simulink model "playground"  (R2024a)
settings: Solver=VariableStepAuto  StartTime=0.0  StopTime=10.0  RelTol=1e-3
InitFcn:
  | a = 0.672; % M + ma/2 + mb, kg
  | b = 0.0051; % (ma/2 + mb)*L, kg*m
  | % c = 0.0021; % (ma/4 + mb)*L^2 + I, kg*m^2
  | g = 9.81;
  | u = 1;
  | 
  | T1 = 0.2;
  | T2 = 0.1;
  | Tf = 0.05;
  | 
  | x1 = 0;
  | x2 = 0;
  | x3 = 0;
  | x4 = 0;
  | x1p = 0;
  | x2p = 0;
  | x3p = 0;
  | x4p = 0;
  | 
  | r = 1;
  | 
  | b0 = 1;
  | A = [0 1 0;
  |      0 0 1;
  |      0 0 0];
  | b_ = [0; b0; 0];
  | c = [1; 0; 0];
  | 
  | % A_CP = [0 1;
  | %        0 0];
  | %
  | % b_CP = [0; 1];
  | %
  | % w_CL = 70;
  | %
  | % k = place(A_CP', b_CP, -w_CL*[1 1.01])';
  | %
  | % k_ESO = 0.9;
  | %
  | % l = place(A',c,-w_CL*k_ESO*[0.99,1,1.01])';
  | 
  | % k_ESO = 10;
  | 
  | % wc_ = 70;
  | % Kx_ = place(A',b_,-wc_*[1 1])';
  | %
  | % k = [5;5];
  | %
  | % w0 = 60;
  | % l = place(A',c,-w0*[0.99,1,1.01])';
  | 
  | %% Liczenie k
  | w_CL = 5;
  | n=2;
  | k = zeros(n,1);
  | for i = 1:n
  |     k(i) = ((factorial(n))/(factorial(n-i+1)*factorial(i-1)))*w_CL^(n-i+1);
  | end
  | 
  | k_r = [k(2); 1];
  | 
  | %% Liczenie l
  | k_ESO = 50;
  | l = zeros(n+1,1);
  | 
  | for i = 1:n+1
  |     l(i) = (factorial(n+1)/(factorial(n-i+1)*factorial(i)))*(k_ESO)^(i);
  | end
  | 
  | % %% PRZYPISANIE POSZCZEGÓLNYCH L:
  | % l1 = l(1);
  | % l2 = l(2);
  | % %% OKREŚLENIE BETY:
  | % B1 = 3 * k_ESO;
  | % B2 = 3 * k_ESO^2;
  | % B3 = k_ESO^3;
  | 
  | %% W ARTYKULE MADONSKI K,L ODPOWIADA L I B W ARTYKULE JIN H.
  | l1 = k(2);
  | l2 = k(1);
  | 
  | B1 = l(1);
  | B2 = l(2);
  | B3 = l(3);
  | 
  | %% WYZNACZENIE PARAMETRÓW:
  | Kc = (B2 * l2 + B3 * l1)/(b0*(B1 * l1 + B2 + l2));
  | tau_i = (B2 * l2 + B3 * l1)/(B3 * l2);
  | tau_d = (B1 * l2 + B2 * l1 + B3)/(B2 * l2 + B3 * l1);
  | wl = sqrt(B1 * l1 + B2 + l2);
  | zeta_l = (B1 + l1)/(2*sqrt(B1 * l1 + B2 + l2));
  | %% Wzmocnienia regulatora CPID:
  | Kp = Kc;
  | Ki = Kc/tau_i;
  | Kd = Kc * tau_d;
  | 
  | %% NOWE NASTAWY PID
  | % Kp = (k(1)*l(1)+k(2)*l(3))/(b0*(k(2)*l(1)+l(2)+k(1)));
  | % Ki = (k(1)*l(3))/(b0*(k(2)*l(1)+l(2)+k(1)));
  | % Kd = (k(1)*l(1)+k(2)*l(2)+l(3))/(b0*(k(2)*l(1)+l(2)+k(1)));
settings Model: Creator=kubat  LastModifiedBy=kubat

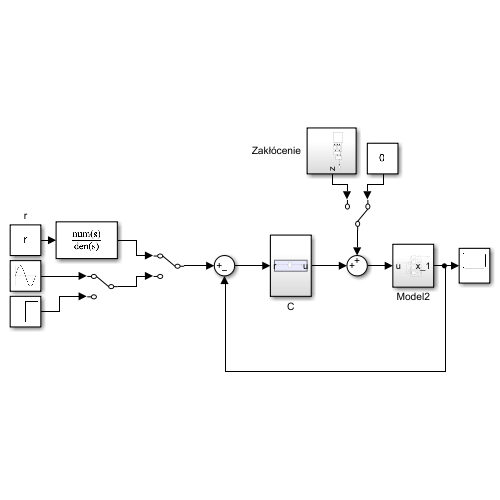
[thumbnail: Simulink's stored preview of the top-level diagram]
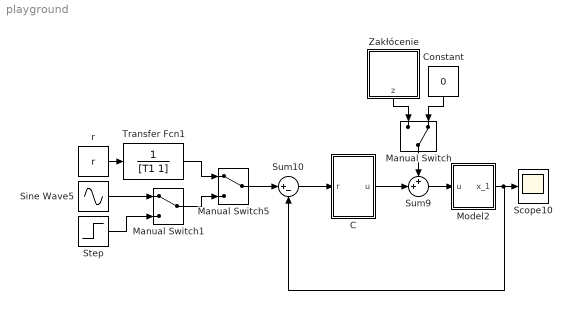
== system playground ==
  C : Subsystem
  Constant : Constant  Value=0
  Manual Switch : ManualSwitch  CurrentSetting=0
  Manual Switch1 : ManualSwitch
  Manual Switch5 : ManualSwitch
  Model2 : Subsystem
  Scope10 : Scope
  Sine Wave5 : Sin  Amplitude=u  SampleTime=0
  Step : Step  After=r  SampleTime=0
  Sum10 : Sum  Inputs=|+-
  Sum9 : Sum  Inputs=++|
  Transfer Fcn1 : TransferFcn  Denominator=[T1 1]
  Zakłócenie : Subsystem
  r : Constant  Value=r
  wires:
  Sum10/1 -> C/1(r)
  Sum9/1 -> Model2/1(u)
  Manual Switch1/1 -> Manual Switch5/2
  Sine Wave5/1 -> Manual Switch1/1
  r/1 -> Transfer Fcn1/1
  Manual Switch5/1 -> Sum10/1
  C/1(u) -> Sum9/2
  Transfer Fcn1/1 -> Manual Switch5/1
  Step/1 -> Manual Switch1/2
  Model2/1(x_1) -> Sum10/2, Scope10/1
  Constant/1 -> Manual Switch/2
  Zakłócenie/1(z) -> Manual Switch/1
  Manual Switch/1 -> Sum9/1

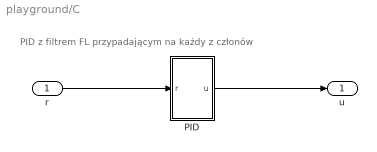
== system playground/C ==
  note: PID z filtrem FL przypadającym na każdy z członów
  r : Inport
  PID : Subsystem
  u : Outport
  wires:
  r/1 -> PID/1(r)
  PID/1(u) -> u/1

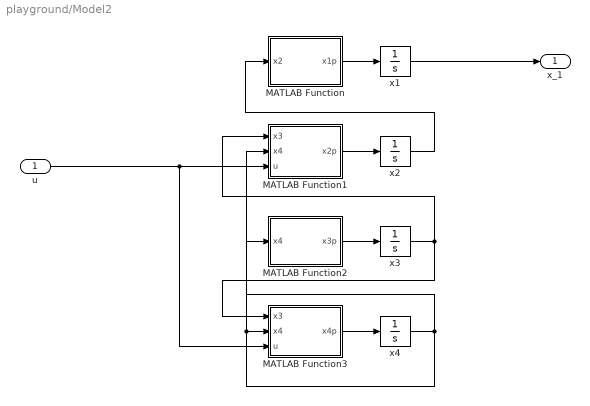
== system playground/Model2 ==
  u : Inport
  MATLAB Function : MATLAB Function  TreatAsAtomicUnit=on
  MATLAB Function1 : MATLAB Function  TreatAsAtomicUnit=on
  MATLAB Function2 : MATLAB Function  TreatAsAtomicUnit=on
  MATLAB Function3 : MATLAB Function  TreatAsAtomicUnit=on
  x{1..4} (4 alike) : Integrator
  x_1 : Outport
  wires:
  u/1 -> MATLAB Function3/3(u), MATLAB Function1/3(u)
  x4/1 -> MATLAB Function2/1(x4), MATLAB Function3/2(x4), MATLAB Function1/2(x4)
  MATLAB Function/1(x1p) -> x1/1
  x3/1 -> MATLAB Function1/1(x3), MATLAB Function3/1(x3)
  x2/1 -> MATLAB Function/1(x2)
  MATLAB Function2/1(x3p) -> x3/1
  MATLAB Function1/1(x2p) -> x2/1
  MATLAB Function3/1(x4p) -> x4/1
  x1/1 -> x_1/1

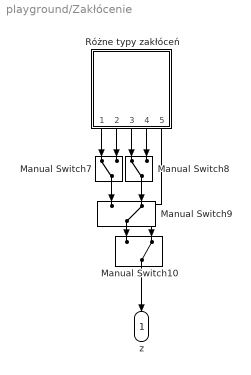
== system playground/Zakłócenie ==
  Manual Switch10 : ManualSwitch  CurrentSetting=0
  Manual Switch7 : ManualSwitch
  Manual Switch8 : ManualSwitch
  Manual Switch9 : ManualSwitch  CurrentSetting=0
  Różne typy zakłóceń : Subsystem
  z : Outport
  wires:
  Manual Switch10/1 -> z/1
  Manual Switch9/1 -> Manual Switch10/1
  Różne typy zakłóceń/2(Const.2) -> Manual Switch7/2
  Różne typy zakłóceń/5(PWM) -> Manual Switch10/2
  Różne typy zakłóceń/4(nSin.) -> Manual Switch8/2
  Różne typy zakłóceń/1(Const.1) -> Manual Switch7/1
  Manual Switch8/1 -> Manual Switch9/2
  Manual Switch7/1 -> Manual Switch9/1
  Różne typy zakłóceń/3(Sin.1) -> Manual Switch8/1

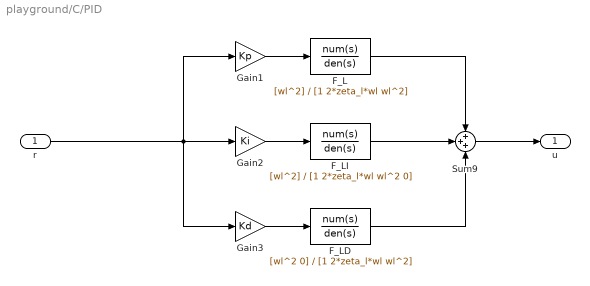
== system playground/C/PID ==
  r : Inport
  F_L : TransferFcn  Numerator=[wl^2]  Denominator=[1 2*zeta_l*wl wl^2]
  F_LD : TransferFcn  Numerator=[wl^2 0]  Denominator=[1 2*zeta_l*wl wl^2]
  F_LI : TransferFcn  Numerator=[wl^2]  Denominator=[1 2*zeta_l*wl wl^2 0]
  Gain1 : Gain  Gain=Kp
  Gain2 : Gain  Gain=Ki
  Gain3 : Gain  Gain=Kd
  Sum9 : Sum  Inputs=+++
  u : Outport
  wires:
  Gain1/1 -> F_L/1
  r/1 -> Gain3/1, Gain2/1, Gain1/1
  Sum9/1 -> u/1
  F_L/1 -> Sum9/1
  Gain2/1 -> F_LI/1
  F_LI/1 -> Sum9/2
  Gain3/1 -> F_LD/1
  F_LD/1 -> Sum9/3

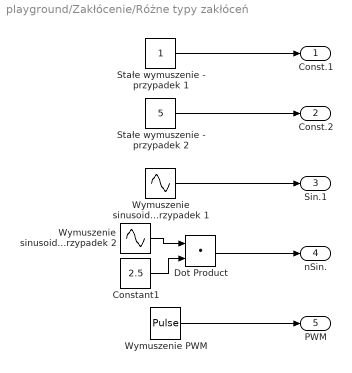
== system playground/Zakłócenie/Różne typy zakłóceń ==
  Constant1 : Constant  Value=2.5
  Dot Product : DotProduct  OutDataTypeStr=Inherit: Inherit via internal rule
  Stałe wymuszenie - przypadek 1 : Constant
  Stałe wymuszenie - przypadek 2 : Constant  Value=5
  "Wymuszenie PWM " : DiscretePulseGenerator  PulseType=Time based  Period=10  PulseWidth=5
  Wymuszenie sinusoidalne - przypadek 1 : Sin  Amplitude=u  SampleTime=0
  Wymuszenie sinusoidalne - przypadek 2 : Sin  Amplitude=u  SampleTime=0
  Const.1 : Outport
  Const.2 : Outport  Port=2
  Sin.1 : Outport  Port=3
  nSin. : Outport  Port=4
  PWM : Outport  Port=5
  wires:
  Wymuszenie sinusoidalne - przypadek 2/1 -> Dot Product/1
  Constant1/1 -> Dot Product/2
  Stałe wymuszenie - przypadek 1/1 -> Const.1/1
  Wymuszenie sinusoidalne - przypadek 1/1 -> Sin.1/1
  "Wymuszenie PWM "/1 -> PWM/1
  Stałe wymuszenie - przypadek 2/1 -> Const.2/1
  Dot Product/1 -> nSin./1

== matlab function playground/Model2/MATLAB Function ==
  data: x2 input; x1p output
function x1p = fcn(x2)

x1p = x2;

== matlab function playground/Model2/MATLAB Function1 ==
  data: x3 input; x2p output; x4 input; u input
function x2p = fcn(x3, x4,u)
g = 9.81;
a = 0.672;
b = 0.0051;
c_ = 0.0021;
x2p = (((c_/a)/(c_-(b^2/a)*(cos(x3))^2))*u)-((((b^2)/a)*g*sin(x3)*cos(x3))-((c_*b)/a)*sin(x3)*x4^2)/(c_-((b^2/a)*cos(x3)*cos(x3)));

== matlab function playground/Model2/MATLAB Function2 ==
  data: x4 input; x3p output
function x3p = fcn(x4)

x3p = x4;

== matlab function playground/Model2/MATLAB Function3 ==
  data: x3 input; x4 input; x4p output; u input
function x4p = fcn(x3,x4,u)
g = 9.81;
g = 9.81;
a = 0.672;
b = 0.0051;
c_ = 0.0021;
x4p = ((((-b/a)*cos(x3))/(c_-(b^2/a)*cos(x3)^2))*u)+(((-b^2/a)*cos(x3)*sin(x3)*x4^2+b*g*sin(x3))/(c_-(b^2/a)*cos(x3)*cos(x3)));
